simulink model "slsf_buck_org"  (Simulink 10.0)
settings: Solver=ode45  StartTime=0.0  StopTime=Tmax  RelTol=1e-6  EnableMultiTasking=on
undefined symbols (not defined in the file): a00c, a00o, a01c, a01o, a10c, a10o, a11c, a11o, b0c, b0o, b1c, b1o, D, i0, T, v0, Vs, Vs_noise
settings Model: Creator=Omar  LastModifiedBy=bhisma
settings SolverCC: ZeroCrossControl=EnableAll
settings DataIOCC: LimitDataPoints=on  SignalLoggingSaveFormat=ModelDataLogs
settings OptimizationCC: ExpressionDepthLimit=2147483647
settings DebuggingCC: SolverPrmCheckMsg=warning  MultiTaskDSMMsg=warning  MultiTaskCondExecSysMsg=none  StateNameClashWarn=warning
settings GRTTargetCC: GeneratePreprocessorConditionals=Disable all  CombineOutputUpdateFcns=on  GRTInterface=off
settings ConfigComp: CovExternalEMLEnable=off

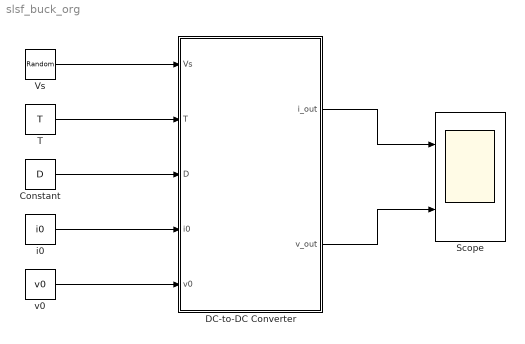
== system slsf_buck_org ==
  Constant : Constant  Value=D
  DC-to-DC Converter : Stateflow chart  TreatAsAtomicUnit=on
  Scope : Scope  NumInputPorts=2
  T : Constant  Value=T
  Vs : RandomNumber  Mean=Vs  Variance=Vs_noise  SampleTime=T/10
  i0 : Constant  Value=i0
  v0 : Constant  Value=v0
  wires:
  T/1 -> DC-to-DC Converter/2(T)
  Vs/1 -> DC-to-DC Converter/1(Vs)
  i0/1 -> DC-to-DC Converter/4(i0)
  v0/1 -> DC-to-DC Converter/5(v0)
  Constant/1 -> DC-to-DC Converter/3(D)
  DC-to-DC Converter/1(i_out) -> Scope/1
  DC-to-DC Converter/2(v_out) -> Scope/2

== stateflow chart DC-to-DC Converter ==
  settings: updateMethod=CONTINUOUS
  state Discontinuous
    du:
    i_dot = a00d*i+a01d*v+b0d*Vs;
    v_dot = a10d*i+a11d*v+b1d*Vs;
    t_dot = 1;
    i_out =i;
    v_out = v;
  state Charging
    du:
    i_dot = a00c*i+a01c*v+b0c*Vs;
    v_dot = a10c*i+a11c*v+b1c*Vs;
    t_dot = 1;
    i_out = i;
    v_out = v;
  state Discharging
    du:
    i_dot = a00o*i+a01o*v+b0o*Vs;
    v_dot = a10o*i+a11o*v+b1o*Vs;
    t_dot = 1;
    i_out = i;
    v_out = v;
  Discharging -> Discontinuous [order 2] : [i<=0]
  Discontinuous -> Charging : [t>= (1-D)*T]
      | {t= 0;}
  Charging -> Discharging : [t>= D*T]
      | {t= 0;}
  Discharging -> Charging [order 1] : [t>= (1-D)*T]
      | {t= 0;}
  (default) -> Charging : {i = i0;
      | v = v0;}
  data: t local double; i local double; a00o local double =a00o; Vs input double =120; T input double; D input double =D; a01o local double =a01o; a10o local double =a10o; a11o local double =a11o; a00c local double =a00c; a01c local double =a01c; a10c local double =a10c; a11c local double =a11c; b0o local double =b0o; b1o local double =b1o; b0c local double =b0c; b1c local double =b1c; v local double; i0 input double; v0 input double; a01d local double; a10d local double; a11d local double; a00d local double; b0d local double; b1d local double; i_out output double; v_out output double
  data t settings: updateMethod=SF_CONTINUOUS_TIME_DATA
  data i settings: updateMethod=SF_CONTINUOUS_TIME_DATA
  data v settings: updateMethod=SF_CONTINUOUS_TIME_DATA
